simulink model "Phase1_Controller"  (R2025b)
settings: Solver=VariableStepAuto  StartTime=0.0  StopTime=10.0  MaxStep=1e-2  RelTol=1e-5
values from neighbouring files (symbols this model uses):
  D_friction = 2    [variables.mat]
  I_joint = 0.5    [variables.mat]
  I_link = 0.15    [variables.mat]
  K_limit = 1.0471975512    [variables.mat]
  L_com = 0.3    [variables.mat]
  m_link = 2    [variables.mat]
  ml_command_age = 20    [variables.mat]
  rate_max = 200    [variables.mat]
  t_gravity_load = 5    [variables.mat]
  thetha_max_soft = 85    [variables.mat]
  thetha_min_soft = 5    [variables.mat]
  torque_max = 30    [variables.mat]
libraries: simulink_extras x3
settings Model: Creator=ranica  LastModifiedBy=adwit

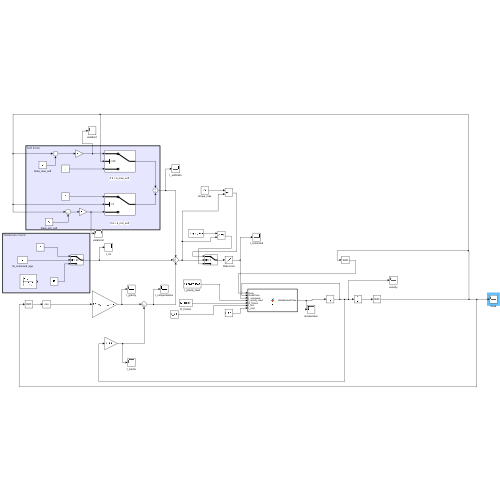
[thumbnail: Simulink's stored preview of the top-level diagram]
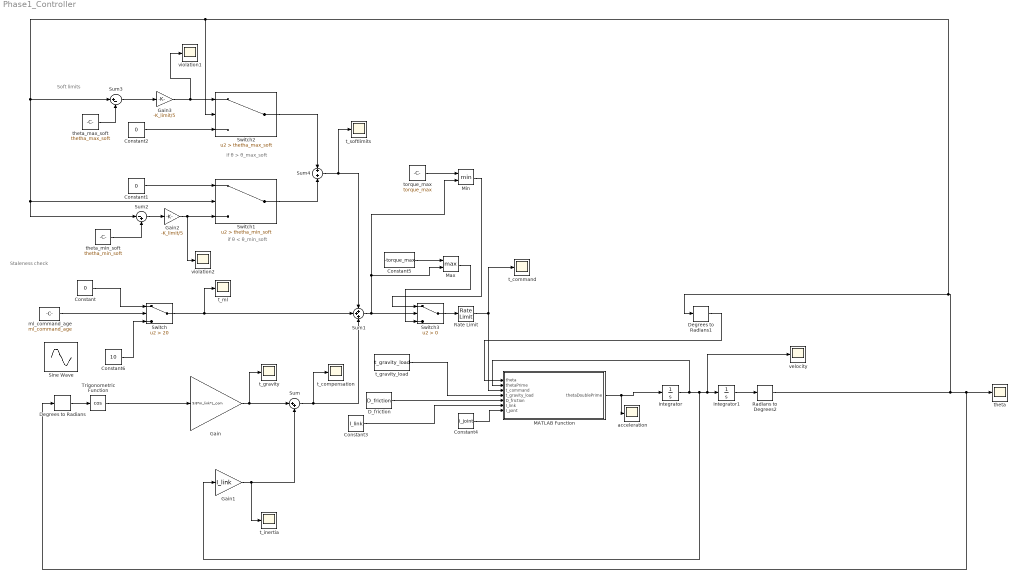
== system Phase1_Controller ==
  note: Soft limits
  note: Staleness check
  note: if θ > θ_max_soft
  note: if θ < θ_min_soft
  Constant : Constant  Value=0
  Constant1 : Constant  Value=0
  Constant2 : Constant  Value=0
  Constant3 : Constant  Value=I_link
  Constant4 : Constant  Value=I_joint
  Constant5 : Constant  Value=-torque_max
  Constant6 : Constant  Value=10
  D_friction : Constant  Value=D_friction
  Degrees to Radians : simulink_extras/Transformations/Degrees to Radians
  Degrees to Radians1 : simulink_extras/Transformations/Degrees to Radians
  Gain : Gain  Gain=9.8*m_link*L_com
  Gain1 : Gain  Gain=I_link
  Gain2 : Gain  Gain=-K_limit/5
  Gain3 : Gain  Gain=-K_limit/5
  Integrator : Integrator
  Integrator1 : Integrator
  MATLAB Function : MATLAB Function  TreatAsAtomicUnit=on
  Max : MinMax  Function=max  Inputs=2
  Min : MinMax  Inputs=2
  Radians to Degrees2 : simulink_extras/Transformations/Radians to Degrees
  Rate Limit : RateLimiter  RisingSlewLimit=rate_max  FallingSlewLimit=-rate_max
  Sine Wave : Sin  Frequency=100  SampleTime=0
  Sum : Sum  Inputs=|++
  Sum1 : Sum  Inputs=+++
  Sum2 : Sum  Inputs=|-+
  Sum3 : Sum  Inputs=|+-
  Sum4 : Sum  Inputs=+|+
  Switch : Switch  Criteria=u2 > Threshold  Threshold=20  SaturateOnIntegerOverflow=off  InputSameDT=off
  Switch1 : Switch  Criteria=u2 > Threshold  Threshold=thetha_min_soft  SaturateOnIntegerOverflow=off  InputSameDT=off
  Switch2 : Switch  Criteria=u2 > Threshold  Threshold=thetha_max_soft  SaturateOnIntegerOverflow=off  InputSameDT=off
  Switch3 : Switch  Criteria=u2 > Threshold  SaturateOnIntegerOverflow=off  InputSameDT=off
  Trigonometric Function : Trigonometry  Operator=cos
  acceleration : Scope
      settings: ActiveDisplayYMinimum=-12.005112001641191  ActiveDisplayYMaximum=9.3254253074565  DataLoggingVariableName=ScopeData8
  ml_command_age : Constant  Value=ml_command_age
  t_command : Scope
      settings: ActiveDisplayYMinimum=-67.037631075120714  ActiveDisplayYMaximum=23.152663920577332
  t_compensation : Scope
      settings: ActiveDisplayYMinimum=-14.864667972880072  ActiveDisplayYMaximum=15.530356100789213  DataLoggingVariableName=ScopeData3
  t_gravity : Scope
      settings: ActiveDisplayYMinimum=-1  ActiveDisplayYMaximum=1
  t_gravity_load : Constant  Value=t_gravity_load
  t_inertia : Scope
      settings: ActiveDisplayYMinimum=-3.5397441265750205  ActiveDisplayYMaximum=3.1235022193721917  DataLoggingVariableName=ScopeData2
  t_ml : Scope
      settings: ActiveDisplayYMinimum=-18.973686746484955  ActiveDisplayYMaximum=13.453115669678192  DataLoggingVariableName=ScopeData4
  t_softlimits : Scope
      settings: ActiveDisplayYMinimum=-9.95804756004255  ActiveDisplayYMaximum=1.1064497288936164  DataLoggingVariableName=ScopeData5
  theta : Scope
      settings: ActiveDisplayYMinimum=110.80449413373488  ActiveDisplayYMaximum=133.48900367563502  DataLoggingVariableName=ScopeData6
  theta_max_soft : Constant  Value=thetha_max_soft
  theta_min_soft : Constant  Value=thetha_min_soft
  torque_max : Constant  Value=torque_max
  velocity : Scope
      settings: ActiveDisplayYMinimum=-2.8920080361743392  ActiveDisplayYMaximum=3.2990674598766465  DataLoggingVariableName=ScopeData7
  violation1 : Scope
      settings: ActiveDisplayYMinimum=-1  ActiveDisplayYMaximum=1
  violation2 : Scope
      settings: ActiveDisplayYMinimum=-20.684449958102746  ActiveDisplayYMaximum=40.96676466137135  DataLoggingVariableName=ScopeData2
  wires:
  ml_command_age/1 -> Switch/2
  Gain/1 -> t_gravity/1, Sum/1
  Gain1/1 -> Sum/2, t_inertia/1
  Sum/1 -> Sum1/3, t_compensation/1
  Switch/1 -> t_ml/1, Sum1/2
  Constant1/1 -> Switch1/1
  theta_min_soft/1 -> Sum2/2
  Sum2/1 -> Gain2/1
  Constant2/1 -> Switch2/3
  Gain3/1 -> violation1/1, Switch2/1
  theta_max_soft/1 -> Sum3/2
  Sum3/1 -> Gain3/1
  Switch2/1 -> Sum4/1
  Sum4/1 -> t_softlimits/1, Sum1/1
  Switch1/1 -> Sum4/2
  MATLAB Function/1(thetaDoublePrime) -> acceleration/1, Integrator/1
  torque_max/1 -> Min/1
  Rate Limit/1 -> t_command/1, MATLAB Function/3(t_command)
  Gain2/1 -> Switch1/3, violation2/1
  t_gravity_load/1 -> MATLAB Function/4(t_gravity_load)
  D_friction/1 -> MATLAB Function/5(D_friction)
  Constant3/1 -> MATLAB Function/6(I_link)
  Constant4/1 -> MATLAB Function/7(I_joint)
  Constant/1 -> Switch/1
  Trigonometric Function/1 -> Gain/1
  Integrator1/1 -> Radians to Degrees2/1
  Degrees to Radians/1 -> Trigonometric Function/1
  Sum1/1 -> Max/2, Min/2, Switch3/2
  Switch3/1 -> Rate Limit/1
  Constant5/1 -> Max/1
  Max/1 -> Switch3/3
  Min/1 -> Switch3/1
  Degrees to Radians1/1 -> MATLAB Function/1(theta)
  Integrator/1 -> MATLAB Function/2(thetaPrime), velocity/1, Integrator1/1, Gain1/1
  Radians to Degrees2/1 -> Switch2/2, Switch1/2, Sum2/1, Sum3/1, Degrees to Radians1/1, Degrees to Radians/1, theta/1
  Constant6/1 -> Switch/3

== matlab function Phase1_Controller/MATLAB Function ==
  data: theta input; thetaDoublePrime output; thetaPrime input; t_command input; t_gravity_load input; D_friction input; I_link input; I_joint input
function thetaDoublePrime = fnc(theta, thetaPrime, t_command, t_gravity_load, D_friction, I_link, I_joint)

thetaDoublePrime = ((t_command - t_gravity_load - D_friction*thetaPrime)) / (I_link + I_joint);
